simulink model "pll03"  (Simulink 8.1)
settings: Solver=ode45  StartTime=0.0  StopTime=10  MaxStep=0.0001  RelTol=1e-3
values from neighbouring files (symbols this model uses):
  delay_t = 0.1:0.05:0.65    [nw_pll01.m]    (also in pll3.m = 0.3; pll5.m)
undefined symbols (not defined in the file or in its folder): fdesignblkfcn, gcbh
libraries: commsynccomp2 x1, commnoisgen2 x1, simulink x1
settings Model: Creator=my88899  LastModifiedBy=my88899
settings DataIOCC: SignalLoggingSaveFormat=Dataset
settings OptimizationCC: ExpressionDepthLimit=128
settings DebuggingCC: FcnCallInpInsideContextMsg=EnableAllAsError
settings GRTTargetCC: CombineOutputUpdateFcns=on  GRTInterface=off

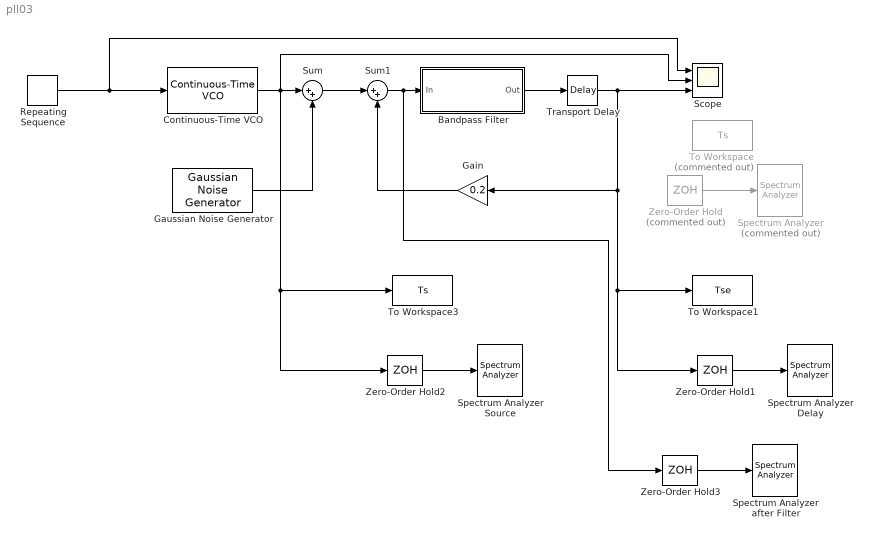
== system pll03 ==
  Bandpass Filter : Subsystem  DialogController=fdesignblkfcn  DialogControllerArgs=DataTag1  InitFcn=fdesignblkfcn(gcbh, {'InitFcn'});  mask(Bandpass Filter){}
      mask help: Design a bandpass filter
      settings: CopyFcn=fdesignblkfcn(gcbh, {'CopyFcn'});
      mask Help: helpview(mapfilelocation('dsp'), 'dspbandpassfilter');
      mask Display: disp('Bandpass');
  Continuous-Time VCO : commsynccomp2/Continuous-Time VCO  Ac=5  Fc=100  Kc=100  Ph=0
  Gain : Gain  Gain=0.2
  Gaussian Noise Generator : commnoisgen2/Gaussian Noise Generator  m=0  d=1  s=2333  Ts=0.1  frameBased=off  sampPerFrame=1  orient=off  outDataType=double
  Repeating Sequence : simulink/Sources/Repeating Sequence  rep_seq_t=[0 1]  rep_seq_y=[0 5]
  Scope : Scope  NumInputPorts=3
      settings: TimeRange=0.1038961038961048  YMin=5.645~-5~-5  YMax=5.7~5~5  MaxDataPoints=100000
  Spectrum Analyzer : SpectrumAnalyzer  Commented=on
      settings: CopyFcn=scopeextensions.ScopeBlock.callback(gcbh, 'onBlockCopy', gcbh);  DeleteFcn=scopeextensions.ScopeBlock.callback(gcbh, 'onBlockDelete');  PreSaveFcn=scopeextensions.ScopeBlock.callback(gcbh, 'onModelSave');  NameChangeFcn=scopeextensions.ScopeBlock.callback(gcbh, 'onBlockRename');  CloseFcn=scopeextensions.ScopeBlock.callback(gcbh, 'onBlockClose');  PreDeleteFcn=scopeextensions.ScopeBlock.callback(gcbh, 'onBlockPreDelete');
  "Spectrum Analyzer Delay " : SpectrumAnalyzer
      settings: CopyFcn=scopeextensions.ScopeBlock.callback(gcbh, 'onBlockCopy', gcbh);  DeleteFcn=scopeextensions.ScopeBlock.callback(gcbh, 'onBlockDelete');  PreSaveFcn=scopeextensions.ScopeBlock.callback(gcbh, 'onModelSave');  NameChangeFcn=scopeextensions.ScopeBlock.callback(gcbh, 'onBlockRename');  CloseFcn=scopeextensions.ScopeBlock.callback(gcbh, 'onBlockClose');  PreDeleteFcn=scopeextensions.ScopeBlock.callback(gcbh, 'onBlockPreDelete');
  "Spectrum Analyzer Source " : SpectrumAnalyzer
      settings: CopyFcn=scopeextensions.ScopeBlock.callback(gcbh, 'onBlockCopy', gcbh);  DeleteFcn=scopeextensions.ScopeBlock.callback(gcbh, 'onBlockDelete');  PreSaveFcn=scopeextensions.ScopeBlock.callback(gcbh, 'onModelSave');  NameChangeFcn=scopeextensions.ScopeBlock.callback(gcbh, 'onBlockRename');  CloseFcn=scopeextensions.ScopeBlock.callback(gcbh, 'onBlockClose');  PreDeleteFcn=scopeextensions.ScopeBlock.callback(gcbh, 'onBlockPreDelete');
  "Spectrum Analyzer after Filter " : SpectrumAnalyzer
      settings: CopyFcn=scopeextensions.ScopeBlock.callback(gcbh, 'onBlockCopy', gcbh);  DeleteFcn=scopeextensions.ScopeBlock.callback(gcbh, 'onBlockDelete');  PreSaveFcn=scopeextensions.ScopeBlock.callback(gcbh, 'onModelSave');  NameChangeFcn=scopeextensions.ScopeBlock.callback(gcbh, 'onBlockRename');  CloseFcn=scopeextensions.ScopeBlock.callback(gcbh, 'onBlockClose');  PreDeleteFcn=scopeextensions.ScopeBlock.callback(gcbh, 'onBlockPreDelete');
  Sum : Sum  Inputs=|++
  Sum1 : Sum  Inputs=|++
  To Workspace : ToWorkspace  Commented=on  VariableName=Ts  SampleTime=-1  SaveFormat=Timeseries
  To Workspace1 : ToWorkspace  VariableName=Tse  SampleTime=-1  SaveFormat=Timeseries
  To Workspace3 : ToWorkspace  VariableName=Ts  SampleTime=-1  SaveFormat=Timeseries
  Transport Delay : TransportDelay  DelayTime=delay_t
  Zero-Order Hold : ZeroOrderHold  Commented=on  SampleTime=0.01
  Zero-Order Hold1 : ZeroOrderHold  SampleTime=0.01
  Zero-Order Hold2 : ZeroOrderHold  SampleTime=0.01
  Zero-Order Hold3 : ZeroOrderHold  SampleTime=0.01
  wires:
  Repeating Sequence/1 -> Scope/1, Continuous-Time VCO/1
  Zero-Order Hold/1 -> Spectrum Analyzer/1
  Gain/1 -> Sum1/2
  Sum/1 -> Sum1/1
  Gaussian Noise Generator/1 -> Sum/2
  Bandpass Filter/1(Out) -> Transport Delay/1
  Zero-Order Hold1/1 -> "Spectrum Analyzer Delay "/1
  Transport Delay/1 -> To Workspace1/1, Zero-Order Hold1/1, Gain/1, Scope/3
  Zero-Order Hold2/1 -> "Spectrum Analyzer Source "/1
  Continuous-Time VCO/1 -> Scope/2, Zero-Order Hold2/1, To Workspace3/1, Sum/1
  Zero-Order Hold3/1 -> "Spectrum Analyzer after Filter "/1
  Sum1/1 -> Zero-Order Hold3/1, Bandpass Filter/1(In)

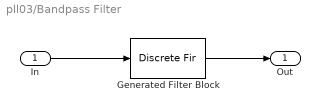
== system pll03/Bandpass Filter ==
  In : Inport
  Generated Filter Block : DiscreteFir  Tag=BlockMethodSubSystem  Coefficients=[0.00044253176381452278 -0.00014197276842491696 -0.00027695473297234958 -0.00048125389204774335 -0.00072274126287417463 -0.00095949738170743662 -0.0011420804272008753 -0.0012189873015733567 -0.0011442966627236836 -0.00088609955061447741 -0.00043410184127011482 0.00019514193189789535 0.00095680641802229531 0.0017807406843933077 0.0025790077401686264 0.0032571052184344651 0.0037273800973886429 0.0039226486657643637 0.0038077144937956409 0.003386716682315819 0.002704726759250895 0.0018428528937446879 0.0009073078457875794 1.3943403761218416e-05 -0.00072927565037796149 -0.0012388808957492089 -0.0014689741062046552 -0.0014183880820097937 -0.0011307201135419209 -0.00068684887910405192 -0.0001908203139989549 0.00024862995490608166 0.00053736452604290078 0.00061246998342990753 0.00044920177121805262 7.3509696391940062e-05 -0.00045192250533183508 -0.0010343824020061744 -0.0015703340224255374 -0.0019649543775457777 -0.0021501890220298847 -0.0020979040300912969 -0.0018255054219785711 -0.0013928483024738822 -0.00089098646398261922 -0.00042468332714599381 -9.2201757618089379e-05 3.4030817604406125e-05 -7.8058078105179148e-05 -0.00041333480341155724 -0.00091174201536752789 -0.0014795128944142802 -0.002007218965461864 -0.0023911892663838674 -0.0025541622464855655 -0.0024610662430619942 -0.0021268079964477712 -0.0016143234053026133 -0.0010229602576875107 -0.00046936375692469668 -6.4387093832159794e-05 0.00010923074940246768 1.3991681677316842e-05 -0.00033384625874321165 -0.00086614141030773577 -0.0014751459255665309 -0.0020342516114814895 -0.002423904065377147 -0.0025536210078045919 -0.0023833043073350256 -0.0019310024982350398 -0.0012713755521700976 -0.00052203528701444889 0.00017904175271108867 0.00070074387209303178 0.00094539440716191552 0.00086931736204450883 0.00049305330701364934 -0.00010095696042055062 -0.00078339713971867849 -0.0014028194030018433 -0.0018156445652749895 -0.0019153804692472714 -0.0016551286317364048 -0.0010587532821282805 -0.00021811358447275332 0.00072349378603989666 0.0015987376727507985 0.0022493384722828014 0.0025582414405049495 0.0024743772799018923 0.0020248275547679979 0.0013115297136403054 0.00049288765971888695 -0.00024662761470622133 -0.0007330850748696043 -0.00083864799419541749 -0.00050876513728120843 0.00022466173495386371 0.0012469917822339849 0.002381088576170501 0.003422116645722876 0.0041769464118569495 0.004504269095299579 0.0043443076044401363 0.0037333851188362491 0.0027994715803452658 0.0017390602367300064 0.00077949097572574584 0.00013386690180229561 -4.2606254337690155e-05 0.00031419768442118807 0.0011613222765592339 0.0023540720414321295 0.0036719238396217624 0.0048606268110912686 0.0056825108043139817 0.0059650193002725163 0.0056376468466623067 0.0047494456166338427 0.0034629207372490101 0.0020248367785422865 0.000719012709292735 -0.00018991560614844914 -0.0005107255474805229 -0.00016684253950480915 0.00078432594813159851 0.0021584366162020175 0.0036771213649391672 0.0050210207047000745 0.0058930114247531182 0.0060791692208563052 0.0054948989374128043 0.0042064297663422226 0.0024232629864873851 0.00046027895450488214 -0.0013216943843816983 -0.0025874856638666874 -0.0030963140489877429 -0.0027540341933841965 -0.0016376887656341437 1.3637384087938527e-05 0.0018410559162068327 0.0034338827088790875 0.0044108926889442615 0.0044985668261790261 0.0035909576091258588 0.0017778724304000166 -0.00066526432427489496 -0.0033254047484540931 -0.0057296845572690413 -0.0074385468538383272 -0.0081360775791033749 -0.0076992808765775755 -0.0062314021253218567 -0.0040510930570941258 -0.0016376096672576824 0.00045883539321044006 0.0017251139639146715 0.0017909024685965353 0.00051062273766540388 -0.0019959377892128207 -0.0053544540757572605 -0.0089985948065020374 -0.012274314056490718 -0.014567282416018415 -0.015429104809636942 -0.01467664542444211 -0.012444288885286895 -0.0091747349931542155 -0.0055480401357097201 -0.0023587739142718576 -0.00036298890763044472 -0.00012349242036681192 -0.0018838960763669613 ...(+5280 chars)]  InputProcessing=Columns as channels (frame based)
  Out : Outport
  wires:
  In/1 -> Generated Filter Block/1
  Generated Filter Block/1 -> Out/1
